simulink model "self_excited_induction_generator"  (R2014b)
settings: Solver=ode23tb  StartTime=0.0  StopTime=10.0  MaxStep=1e-4  RelTol=1e-3
libraries: powerlib x10, powerlib_meascontrol x1
settings Model: Creator=Amr Saleh  LastModifiedBy=Amr Saleh

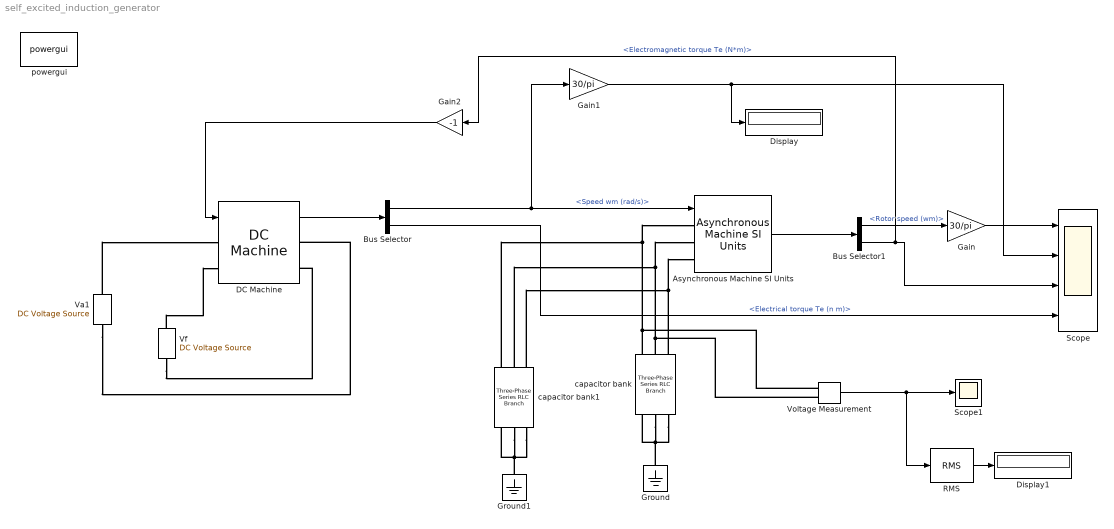
== system self_excited_induction_generator ==
  Asynchronous Machine SI Units : powerlib/Machines/Asynchronous Machine SI Units  PresetModel="15:  5.4 HP (4KW)   400 V  50Hz 1430 RPM"  MechanicalLoad=Speed w  ShowDetailedParameters=on  RotorType=Squirrel-cage  ReferenceFrame=Stationary  Units=SI  MeasurementBus=off  NominalParameters=[4000 400 50]  Stator=[1.405 0.005839]  Rotor=[1.395 0.005839]  Cage1=[ 0.022 0.226/377]  Cage2=[ 0.022 0.226/377]  Lm=0.1722  Mechanical=[0.0131 0.002985 2]  PolePairs=2  InitialConditions=[1 0 1 1 1 0 -120 120]  SimulateSaturation=off  Saturation=[14.03593122, 27.81365428, 53.79336849, 72.68890987, 97.98006896, 148.6815601, 215.7428561, 302.9841135, 420.4778367 ; 230, 322, 414, 460, 506, 552, 598, 644, 690]  LoadFlowParameters=1492000  TsPowergui=0  TsBlock=-1  IterativeModel=Trapezoidal non iterative  Pmec=0
  Bus Selector : BusSelector  OutputSignals=Speed wm (rad/s),Electrical torque Te (n m)
  Bus Selector1 : BusSelector  OutputSignals=Mechanical.Rotor speed (wm),Mechanical.Electromagnetic torque Te (N*m)
  DC Machine : powerlib/Machines/DC Machine  PresetModel=01: 5HP 240V 1750RPM Field:300V  MechanicalLoad=Torque TL  FieldType=Wound  ShowDetailedParameters=on  MeasurementBus=off  RLa=[2.581 0.028]  RLf=[281.3 156]  Laf=0.9483  MachineConstant=Torque constant (N.m/A)  Ke=1.8  Kt=1.8  J=0.02215  Bm=0.002953  Tf=0.5161  w0=1  Ifinit=1  TsPowergui=0  TsBlock=-1
  Display : Display
  Display1 : Display
  Gain : Gain  Gain=30/pi
  Gain1 : Gain  Gain=30/pi
  Gain2 : Gain  Gain=-1
  Ground : powerlib/Elements/Ground  LConnTagsString=a
  Ground1 : powerlib/Elements/Ground  LConnTagsString=a
  RMS : powerlib_meascontrol/Measurements/RMS  TrueRMS=off  Freq=50  RMSInit=0  Ts=0
  Scope : Scope  NumInputPorts=4
      settings: YMin=1600~1600~-20~0  YMax=2400~2400~0~20
  Scope1 : Scope
      settings: YMin=-800  YMax=800
  Va1 : powerlib/Electrical Sources/DC Voltage Source  Amplitude=240  Measurements=None
  Vf : powerlib/Electrical Sources/DC Voltage Source  Amplitude=300  Measurements=None
  Voltage Measurement : powerlib/Measurements/Voltage Measurement  PhasorSimulation=off  OutputType=Complex  PSBequivalent=0
  capacitor bank : powerlib/Elements/Three-Phase Series RLC Branch  LConnTagsString=A|B|C  RConnTagsString=A|B|C  BranchType=C  Resistance=1  Inductance=1e-3  Capacitance=54e-6  Measurements=None
  capacitor bank1 : powerlib/Elements/Three-Phase Series RLC Branch  LConnTagsString=A|B|C  RConnTagsString=A|B|C  BranchType=R  Resistance=50  Inductance=1e-3  Capacitance=100e-6  Measurements=None
  powergui : powerlib/powergui  Priority=1  SimulationMode=Continuous  SolverType=Tustin/Backward Euler (TBE)  SampleTime=50e-6  frequency=60  SPID=off  DisableSnubberDevices=off  DisableRonSwitches=off  DisableVfSwitches=off  SwTol=0  DisplayEquations=off  Interpol=off  methode=off  Ts=100  frequencyindice=50  Pbase=100e6  ErrMax=1e-4  Iterations=50  UnitsV=kV  UnitsW=MW  FunctionMessages=off  echomessages=off  HookPort=off  EnableUseOfTLC=off  x0status=blocks  RestoreLinks=warning  ResistiveCurrentMeasurement=off  Frange=[0:2:500]  Ylog=off  Xlog=on  ShowGrid=off  save=off  variable=ZData  structure=0  ZoomFFT=off  StartTime=0.0  cycles=1  DisplayStyle=1  fundamental=60  FreqAxis=off  MaxFrequency=1000  frequencyindicesteady=1  RmsSteady=1  display=off
  wires:
  DC Machine/1 -> Bus Selector/1
  Bus Selector/1 -> Gain1/1, Asynchronous Machine SI Units/1  "<Speed wm (rad/s)>"
  Asynchronous Machine SI Units/1 -> Bus Selector1/1
  Bus Selector1/1 -> Gain/1  "<Rotor speed (wm)>"
  Gain/1 -> Scope/1
  Gain1/1 -> Display/1, Scope/2
  Bus Selector1/2 -> Gain2/1, Scope/3  "<Electromagnetic torque Te (N*m)>"
  Bus Selector/2 -> Scope/4  "<Electrical torque Te (n m)>"
  Voltage Measurement/1 -> RMS/1, Scope1/1
  Gain2/1 -> DC Machine/1
  RMS/1 -> Display1/1
  connections:
  Va1/RConn1 -- DC Machine/LConn1
  Va1/LConn1 -- DC Machine/RConn1
  Vf/RConn1 -- DC Machine/LConn2
  Vf/LConn1 -- DC Machine/RConn2
  capacitor bank/RConn3 -- Ground/LConn1 -- capacitor bank/RConn2 -- capacitor bank/RConn1
  capacitor bank/LConn1 -- capacitor bank1/LConn1 -- Asynchronous Machine SI Units/LConn1 -- Voltage Measurement/LConn1
  capacitor bank/LConn2 -- Voltage Measurement/LConn2 -- capacitor bank1/LConn2 -- Asynchronous Machine SI Units/LConn2
  capacitor bank/LConn3 -- capacitor bank1/LConn3 -- Asynchronous Machine SI Units/LConn3
  capacitor bank1/RConn3 -- Ground1/LConn1 -- capacitor bank1/RConn2 -- capacitor bank1/RConn1
